simulink model "MainScheme"  (R2016b)
settings: Solver=VariableStepAuto  StartTime=0.0  StopTime=inf  RelTol=1e-3  EnableMultiTasking=on
libraries: dspvision x2, dspsnks4 x1, dspfdesign x1
settings Model: Creator=Mao_Tony  LastModifiedBy=Odaimoko_
settings OptimizationCC: LifeSpan=inf
settings DebuggingCC: SFUnexpectedBacktrackingDiag=warning  SFNoUnconditionalDefaultTransitionDiag=warning  SFExecutionAtInitializationDiag=none
settings GRTTargetCC: TargetLangStandard=C89/C90 (ANSI)  GeneratePreprocessorConditionals=Disable all
settings ConfigComp: CovMetricSettings=dw  CovHtmlReporting=on  CovSaveCumulativeToWorkspaceVar=on  CovSaveSingleToWorkspaceVar=on  CovExternalEMLEnable=off

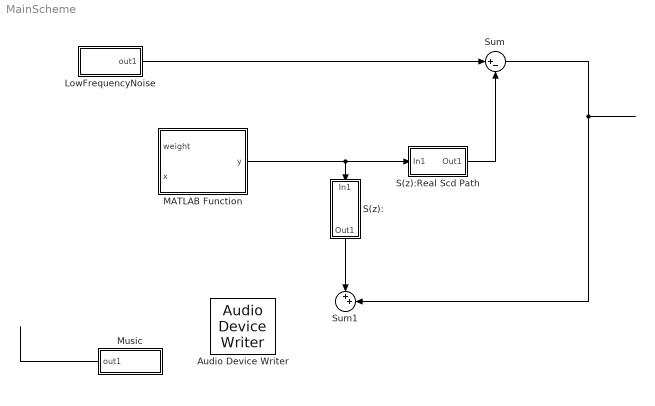
== system MainScheme ==
  Audio Device Writer : dspsnks4/Audio Device Writer  Driver=DirectSound  Device=Default  InheritSampleRate=on  SampleRate=44100  BitDepth=16-bit integer  BufferSize=4096  NumBuffers=10  DefaultOutputChannelMapping=on  OutputChannelMapping=1:2  OutputNumUnderrunSamples=off  DriverIdx=1  DeviceWarnFlag=''
  LowFrequencyNoise : Subsystem
  MATLAB Function : MATLAB Function  Description=W  TreatAsAtomicUnit=on
  Music : Subsystem
  S(z): : Subsystem
  S(z):Real Scd Path : Subsystem
  Sum : Sum  Inputs=|+-
  Sum1 : Sum  Inputs=|++
  wires:
  LowFrequencyNoise/1("out1 ") -> Sum/1
  Sum/1 -> Sum1/2
  Music/1("out1 ") -> ?
  S(z):Real Scd Path/1(Out1) -> Sum/2
  MATLAB Function/1(y) -> S(z):/1(In1), S(z):Real Scd Path/1(In1)
  S(z):/1(Out1) -> Sum1/1

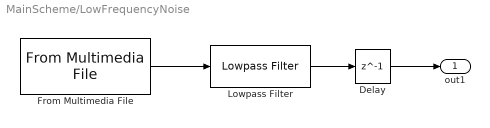
== system MainScheme/LowFrequencyNoise ==
  Delay : Delay  DelayLength=1  InitialCondition=0
  From Multimedia File : dspvision/From Multimedia File  inputFilename=/Users/new/Desktop/NoiseCancelingHeadPhone/Noise.wav  loop=on  numPlays=inf  outputStreams=Audio only  videoDataType=single  audioDataType=double  inheritSampleTime=on  userDefinedSampleTime=1/30  noAudioOutput=off  isIntensityVideo=off  fourcc=RGB  colorVideoFormat=Separate color signals  outputEOF=off  dataOrg=Column-major  audioFrameSize=32  computeAudioFrameSize=off  outSamplingMode=Sample based
  Lowpass Filter : dspfdesign/Lowpass Filter  FilterType=FIR  DesignForMinimumOrder=on  FilterOrder=50  PassbandFrequency=8e2  StopbandFrequency=12e3  PassbandRipple=0.1  StopbandAttenuation=80  InheritSampleRate=off  SampleRate=44100  roundingMode=Floor  coeffsDataTypeStr=fixdt(1,16)  SimulateUsing=Interpreted execution
  "out1 " : Outport
  wires:
  From Multimedia File/1 -> Lowpass Filter/1
  Lowpass Filter/1 -> Delay/1
  Delay/1 -> "out1 "/1

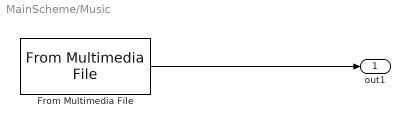
== system MainScheme/Music ==
  From Multimedia File : dspvision/From Multimedia File  inputFilename=/Users/new/Desktop/NoiseCancelingHeadPhone/Music.wav  loop=on  numPlays=inf  outputStreams=Audio only  videoDataType=single  audioDataType=double  inheritSampleTime=on  userDefinedSampleTime=1/30  noAudioOutput=off  isIntensityVideo=off  fourcc=RGB  colorVideoFormat=Separate color signals  outputEOF=off  dataOrg=Column-major  audioFrameSize=32  computeAudioFrameSize=off  outSamplingMode=Sample based
  "out1 " : Outport
  wires:
  From Multimedia File/1 -> "out1 "/1

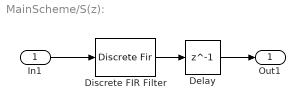
== system MainScheme/S(z): ==
  In1 : Inport
  Delay : Delay  DelayLength=1  InitialCondition=0
  Discrete FIR Filter : DiscreteFir  Coefficients=[0.7 0.5 0.5]
  Out1 : Outport
  wires:
  In1/1 -> Discrete FIR Filter/1
  Discrete FIR Filter/1 -> Delay/1
  Delay/1 -> Out1/1

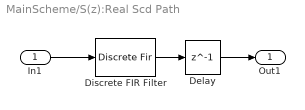
== system MainScheme/S(z):Real Scd Path ==
  In1 : Inport
  Delay : Delay  DelayLength=1  InitialCondition=0
  Discrete FIR Filter : DiscreteFir  Coefficients=[0.7 0.5 0.5]
  Out1 : Outport
  wires:
  In1/1 -> Discrete FIR Filter/1
  Discrete FIR Filter/1 -> Delay/1
  Delay/1 -> Out1/1

== matlab function MainScheme/MATLAB Function ==
  data: weight input; y output; x input
function y = W_FIR_Filter(weight,x)

y = x;
end
